simulink model "CTRL_LO_ST5_test"  (R2023b)
settings: Solver=VariableStepAuto  StartTime=0.0  StopTime=10.0  RelTol=1e-3
libraries: CTRL_LO_ST5 x1
settings Model: Creator=blatak  LastModifiedBy=blatak

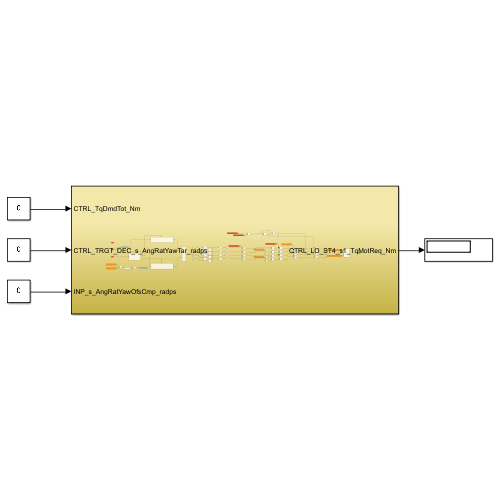
[thumbnail: Simulink's stored preview of the top-level diagram]
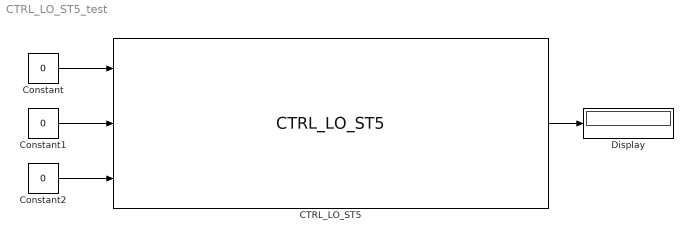
== system CTRL_LO_ST5_test ==
  CTRL_LO_ST5 : CTRL_LO_ST5/CTRL_LO_ST5  SystemSampleTime=-1  VariantActivationTime=update diagram  AllowFlexibleInterface=on  Latency=0  AutoFrameSizeCalculation=off
  Constant : Constant  Value=0  OutDataTypeStr=single
  Constant1 : Constant  Value=0  OutDataTypeStr=single
  Constant2 : Constant  Value=0  OutDataTypeStr=single
  Display : Display
  wires:
  Constant/1 -> CTRL_LO_ST5/1
  Constant1/1 -> CTRL_LO_ST5/2
  Constant2/1 -> CTRL_LO_ST5/3
  CTRL_LO_ST5/1 -> Display/1
